simulink subsystem "Position_PI_C"  (R2022b)
settings: Solver=VariableStepAuto  StartTime=0.0  StopTime=10.0  RelTol=1e-3
undefined symbols (not defined in the file or in its folder): conv, Ri, Rt, Rw, sat
settings Model: Creator=gotta  LastModifiedBy=gotta

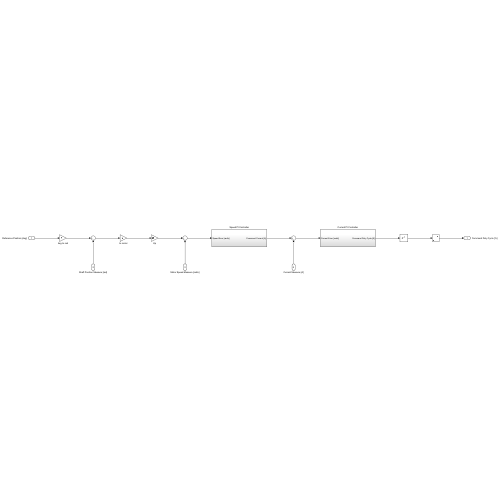
[thumbnail: Simulink's stored preview of the top-level diagram]
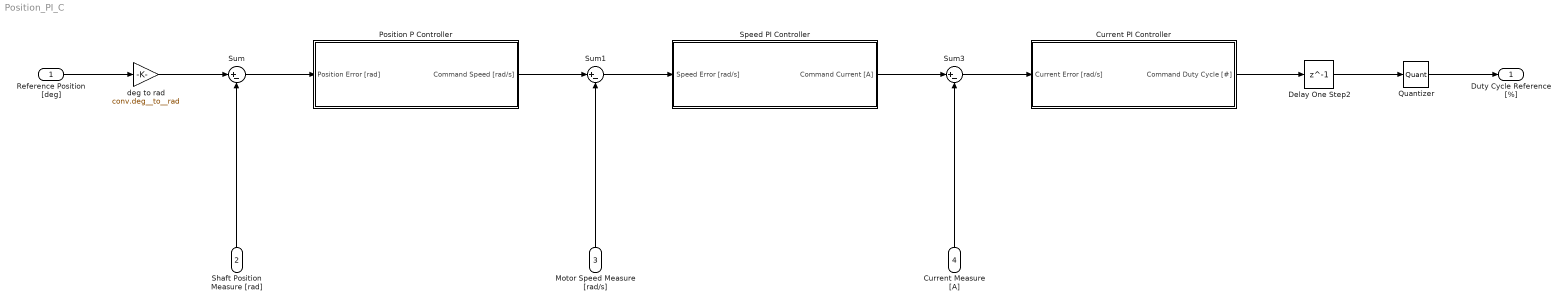
== system Position_PI_C ==
  Reference Position [deg] : Inport
  Shaft Position Measure [rad] : Inport  Port=2
  Motor Speed Measure [rad/s] : Inport  Port=3
  Current Measure [A] : Inport  Port=4
  Current PI Controller : Subsystem
  Delay One Step2 : Delay  DelayLength=1
  Position P Controller : Subsystem
  Quantizer : Quantizer  QuantizationInterval=uc.duty_step
  Speed PI Controller : Subsystem
  Sum : Sum  Inputs=|+-
  Sum1 : Sum  Inputs=|+-
  Sum3 : Sum  Inputs=|+-
  deg to rad : Gain  Gain=conv.deg__to__rad
  Duty Cycle Reference [%] : Outport
  wires:
  Sum1/1 -> Speed PI Controller/1(Speed Error [rad/s])
  Quantizer/1 -> Duty Cycle Reference [%]/1
  Reference Position [deg]/1 -> deg to rad/1
  Current Measure [A]/1 -> Sum3/2
  Motor Speed Measure [rad/s]/1 -> Sum1/2
  Speed PI Controller/1(Command Current [A]) -> Sum3/1
  Sum3/1 -> Current PI Controller/1(Current Error [rad/s])
  Current PI Controller/1(Command Duty Cycle [#]) -> Delay One Step2/1
  Shaft Position Measure [rad]/1 -> Sum/2
  Position P Controller/1(Command Speed [rad/s]) -> Sum1/1
  deg to rad/1 -> Sum/1
  Sum/1 -> Position P Controller/1(Position Error [rad])
  Delay One Step2/1 -> Quantizer/1

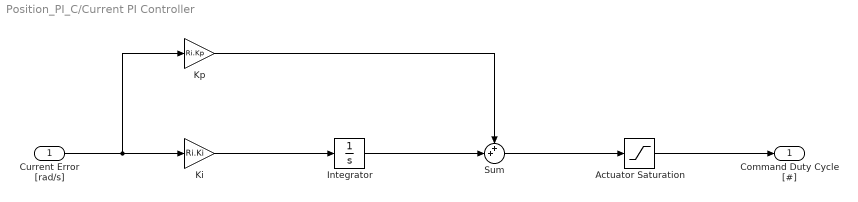
== system Position_PI_C/Current PI Controller ==
  Current Error [rad/s] : Inport
  Actuator Saturation : Saturate  UpperLimit=sat.d  LowerLimit=-sat.d
  Integrator : Integrator  LimitOutput=on  UpperSaturationLimit=sat.d  LowerSaturationLimit=-sat.d
  Ki : Gain  Gain=Ri.Ki
  Kp : Gain  Gain=Ri.Kp
  Sum : Sum  Inputs=++|
  Command Duty Cycle [#] : Outport
  wires:
  Actuator Saturation/1 -> Command Duty Cycle [#]/1
  Current Error [rad/s]/1 -> Kp/1, Ki/1
  Kp/1 -> Sum/1
  Sum/1 -> Actuator Saturation/1
  Ki/1 -> Integrator/1
  Integrator/1 -> Sum/2

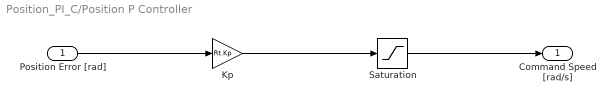
== system Position_PI_C/Position P Controller ==
  Position Error [rad] : Inport
  Kp : Gain  Gain=Rt.Kp
  Saturation : Saturate  UpperLimit=sat.w  LowerLimit=-sat.w
  Command Speed [rad/s] : Outport
  wires:
  Kp/1 -> Saturation/1
  Saturation/1 -> Command Speed [rad/s]/1
  Position Error [rad]/1 -> Kp/1

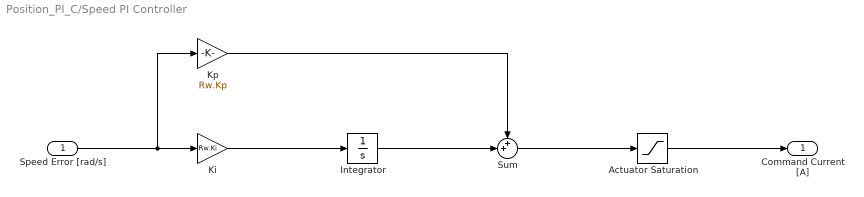
== system Position_PI_C/Speed PI Controller ==
  Speed Error [rad/s] : Inport
  Actuator Saturation : Saturate  UpperLimit=sat.I  LowerLimit=-sat.I
  Integrator : Integrator  LimitOutput=on  UpperSaturationLimit=sat.I  LowerSaturationLimit=-sat.I
  Ki : Gain  Gain=Rw.Ki
  Kp : Gain  Gain=Rw.Kp
  Sum : Sum  Inputs=++|
  Command Current [A] : Outport
  wires:
  Kp/1 -> Sum/1
  Actuator Saturation/1 -> Command Current [A]/1
  Speed Error [rad/s]/1 -> Ki/1, Kp/1
  Sum/1 -> Actuator Saturation/1
  Ki/1 -> Integrator/1
  Integrator/1 -> Sum/2
